simulink model "Loftin_Equations"  (R2023a)
settings: Solver=FixedStepAuto  StartTime=0.0  StopTime=1.0  FixedStep=1.0  RelTol=1e-3
settings Model: Creator=horty  LastModifiedBy=horty

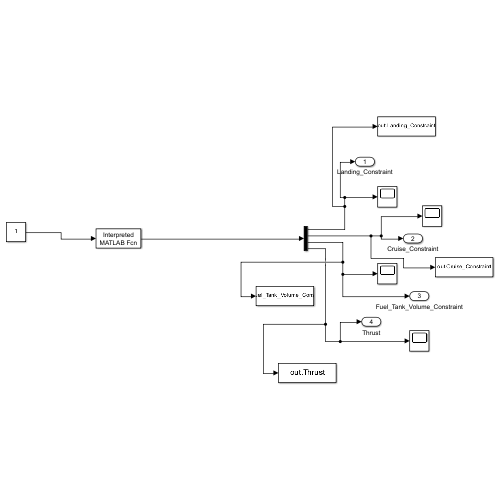
[thumbnail: Simulink's stored preview of the top-level diagram]
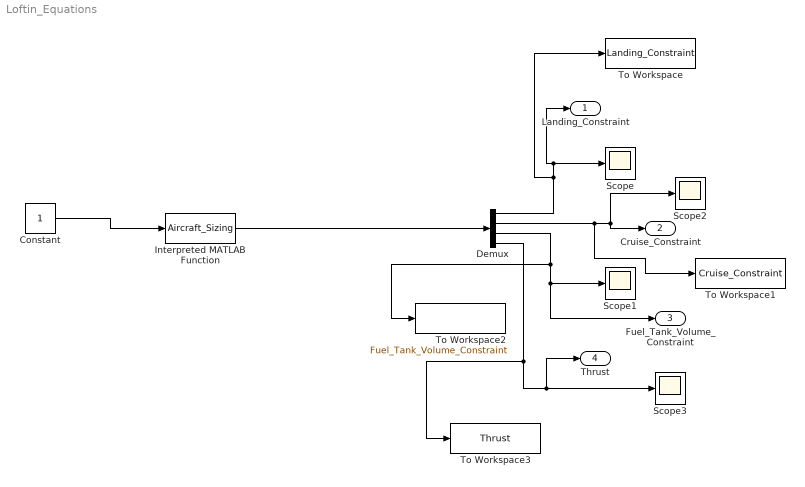
== system Loftin_Equations ==
  Constant : Constant
  Demux : Demux
  Interpreted MATLAB Function : MATLABFcn  MATLABFcn=Aircraft_Sizing  OutputSignalType=real
  Scope{,1..3} (4 alike) : Scope
  To Workspace : ToWorkspace  VariableName=Landing_Constraint  SampleTime=-1
  To Workspace1 : ToWorkspace  VariableName=Cruise_Constraint  SampleTime=-1
  To Workspace2 : ToWorkspace  VariableName=Fuel_Tank_Volume_Constraint  SampleTime=-1
  To Workspace3 : ToWorkspace  VariableName=Thrust  SampleTime=-1
  Landing_Constraint : Outport
  Cruise_Constraint : Outport  Port=2
  Fuel_Tank_Volume_Constraint : Outport  Port=3
  Thrust : Outport  Port=4
  wires:
  Interpreted MATLAB Function/1 -> Demux/1
  Demux/1 -> To Workspace/1, Scope/1, Landing_Constraint/1
  Demux/3 -> To Workspace2/1, Fuel_Tank_Volume_Constraint/1, Scope1/1
  Constant/1 -> Interpreted MATLAB Function/1
  Demux/2 -> To Workspace1/1, Cruise_Constraint/1, Scope2/1
  Demux/4 -> To Workspace3/1, Thrust/1, Scope3/1
